simulink model "nonlinearplanner"  (R2021a)
settings: Solver=VariableStepAuto  StartTime=0.0  StopTime=10.0  RelTol=1e-3
values from neighbouring files (symbols this model uses):
  DELAY_LANDING = 4    [variables.m]
  DERIVATIVE_GAIN = 0.002    [variables.m]
  GAIN_LANDING = 0.0022    [variables.m]
  GAIN_TRACK = 0.0038    [variables.m]
  TIME_HOLD = 0.2    [variables.m]
undefined symbols (not defined in the file or in its folder): Ts
libraries: simulink x2
settings Model: Creator=s2130866  LastModifiedBy=s2130866

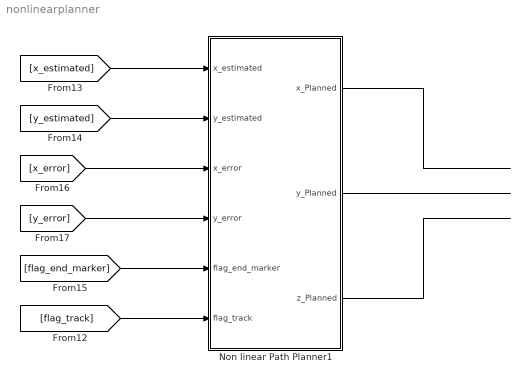
== system nonlinearplanner ==
  Non linear Path Planner1 : Subsystem
  wires:
  Non linear Path Planner1/1(x_Planned) -> ?
  [x_error] -> Non linear Path Planner1/3(x_error)
  Non linear Path Planner1/3(z_Planned) -> ?
  [y_error] -> Non linear Path Planner1/4(y_error)
  [flag_end_marker] -> Non linear Path Planner1/5(flag_end_marker)
  [x_estimated] -> Non linear Path Planner1/1(x_estimated)
  [flag_track] -> Non linear Path Planner1/6(flag_track)
  [y_estimated] -> Non linear Path Planner1/2(y_estimated)
  Non linear Path Planner1/2(y_Planned) -> ?

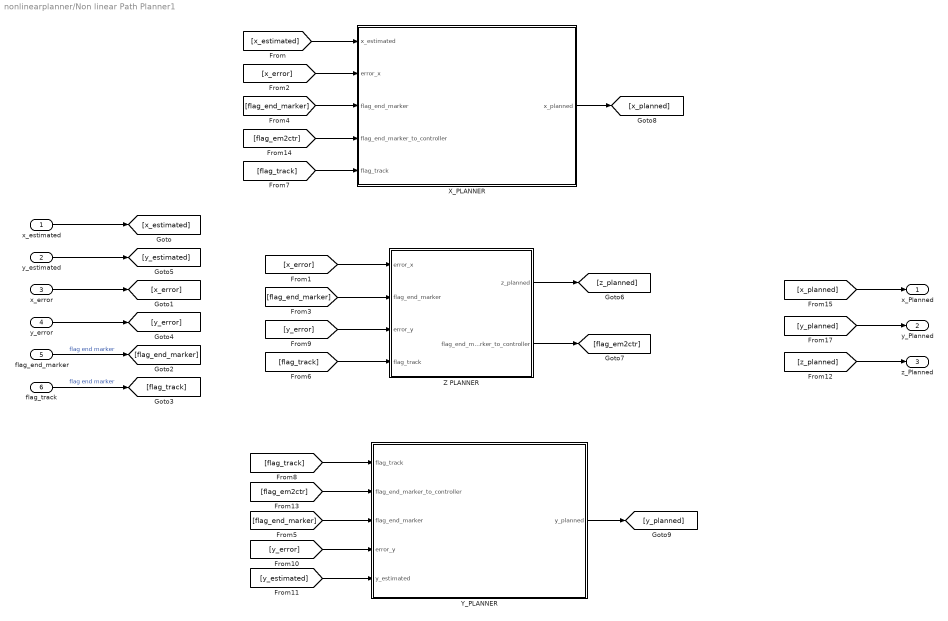
== system nonlinearplanner/Non linear Path Planner1 ==
  x_estimated : Inport
  y_estimated : Inport  Port=2
  x_error : Inport  Port=3
  y_error : Inport  Port=4
  flag_end_marker : Inport  Port=5
  flag_track : Inport  Port=6
  X_PLANNER : Subsystem
  Y_PLANNER : Subsystem
  Z PLANNER : Subsystem
  x_Planned : Outport  VectorParamsAs1DForOutWhenUnconnected=off
  y_Planned : Outport  Port=2  VectorParamsAs1DForOutWhenUnconnected=off
  z_Planned : Outport  Port=3  VectorParamsAs1DForOutWhenUnconnected=off
  wires:
  x_estimated/1 -> [x_estimated]
  [x_estimated] -> X_PLANNER/1(x_estimated)
  x_error/1 -> [x_error]
  [x_error] -> Z PLANNER/1(error_x)
  [x_error] -> X_PLANNER/2(error_x)
  flag_end_marker/1 -> [flag_end_marker]  "flag end marker"
  [flag_end_marker] -> Z PLANNER/2(flag_end_marker)
  [flag_end_marker] -> X_PLANNER/3(flag_end_marker)
  [flag_end_marker] -> Y_PLANNER/3(flag_end_marker)
  flag_track/1 -> [flag_track]  "flag end marker"
  [flag_track] -> Z PLANNER/4(flag_track)
  [flag_track] -> X_PLANNER/5(flag_track)
  [flag_track] -> Y_PLANNER/1(flag_track)
  y_error/1 -> [y_error]
  [y_error] -> Z PLANNER/3(error_y)
  [y_error] -> Y_PLANNER/4(error_y)
  y_estimated/1 -> [y_estimated]
  [y_estimated] -> Y_PLANNER/5(y_estimated)
  [z_planned] -> z_Planned/1
  Z PLANNER/1(z_planned) -> [z_planned]
  Z PLANNER/2(flag_end_marker_to_controller) -> [flag_em2ctr]
  [flag_em2ctr] -> Y_PLANNER/2(flag_end_marker_to_controller)
  [flag_em2ctr] -> X_PLANNER/4(flag_end_marker_to_controller)
  X_PLANNER/1(x_planned) -> [x_planned]
  Y_PLANNER/1(y_planned) -> [y_planned]
  [x_planned] -> x_Planned/1
  [y_planned] -> y_Planned/1

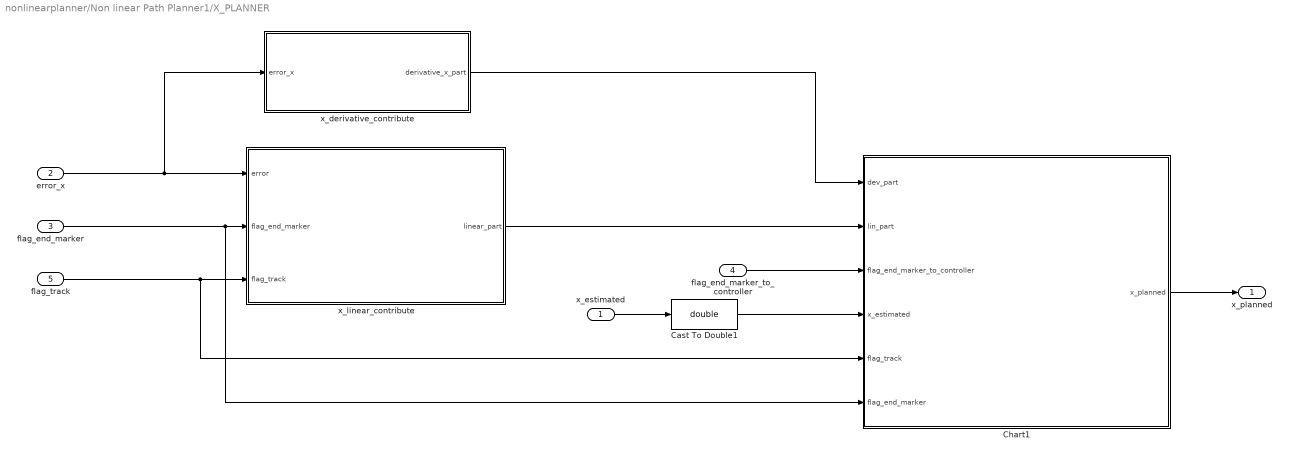
== system nonlinearplanner/Non linear Path Planner1/X_PLANNER ==
  x_estimated : Inport
  error_x : Inport  Port=2
  flag_end_marker : Inport  Port=3
  flag_end_marker_to_controller : Inport  Port=4
  flag_track : Inport  Port=5
  Cast To Double1 : DataTypeConversion  OutDataTypeStr=double
  Chart1 : Stateflow chart  TreatAsAtomicUnit=on
  "x_derivative_contribute " : Subsystem
  x_linear_contribute : Stateflow chart  TreatAsAtomicUnit=on
  x_planned : Outport  VectorParamsAs1DForOutWhenUnconnected=off
  wires:
  "x_derivative_contribute "/1(derivative_x_part) -> Chart1/1(dev_part)
  x_estimated/1 -> Cast To Double1/1
  flag_end_marker_to_controller/1 -> Chart1/3(flag_end_marker_to_controller)
  error_x/1 -> "x_derivative_contribute "/1(error_x), x_linear_contribute/1(error)
  Cast To Double1/1 -> Chart1/4(x_estimated)
  flag_track/1 -> Chart1/5(flag_track), x_linear_contribute/3(flag_track)
  x_linear_contribute/1(linear_part) -> Chart1/2(lin_part)
  flag_end_marker/1 -> Chart1/6(flag_end_marker), x_linear_contribute/2(flag_end_marker)
  Chart1/1(x_planned) -> x_planned/1

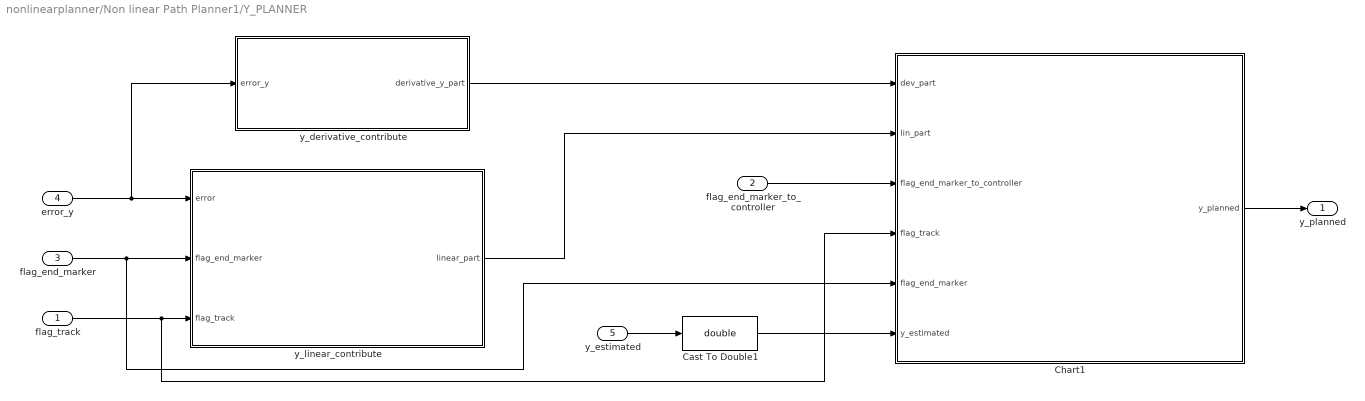
== system nonlinearplanner/Non linear Path Planner1/Y_PLANNER ==
  flag_track : Inport
  flag_end_marker_to_controller : Inport  Port=2
  flag_end_marker : Inport  Port=3
  error_y : Inport  Port=4
  y_estimated : Inport  Port=5
  Cast To Double1 : DataTypeConversion  OutDataTypeStr=double
  Chart1 : Stateflow chart  TreatAsAtomicUnit=on
  "y_derivative_contribute " : Subsystem
  y_linear_contribute : Stateflow chart  TreatAsAtomicUnit=on
  y_planned : Outport  VectorParamsAs1DForOutWhenUnconnected=off
  wires:
  error_y/1 -> y_linear_contribute/1(error), "y_derivative_contribute "/1(error_y)
  "y_derivative_contribute "/1(derivative_y_part) -> Chart1/1(dev_part)
  y_estimated/1 -> Cast To Double1/1
  flag_end_marker/1 -> Chart1/5(flag_end_marker), y_linear_contribute/2(flag_end_marker)
  flag_track/1 -> Chart1/4(flag_track), y_linear_contribute/3(flag_track)
  y_linear_contribute/1(linear_part) -> Chart1/2(lin_part)
  Cast To Double1/1 -> Chart1/6(y_estimated)
  flag_end_marker_to_controller/1 -> Chart1/3(flag_end_marker_to_controller)
  Chart1/1(y_planned) -> y_planned/1

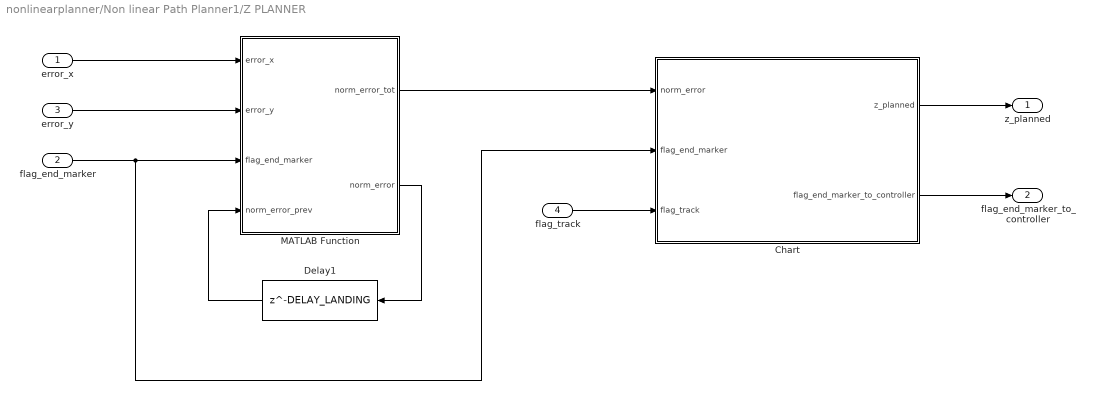
== system nonlinearplanner/Non linear Path Planner1/Z PLANNER ==
  error_x : Inport
  flag_end_marker : Inport  Port=2
  error_y : Inport  Port=3
  flag_track : Inport  Port=4
  Chart : Stateflow chart  TreatAsAtomicUnit=on
  Delay1 : Delay  DelayLength=DELAY_LANDING
  MATLAB Function : MATLAB Function  TreatAsAtomicUnit=on
  z_planned : Outport  VectorParamsAs1DForOutWhenUnconnected=off
  flag_end_marker_to_controller : Outport  Port=2  VectorParamsAs1DForOutWhenUnconnected=off
  wires:
  error_y/1 -> MATLAB Function/2(error_y)
  error_x/1 -> MATLAB Function/1(error_x)
  flag_end_marker/1 -> Chart/2(flag_end_marker), MATLAB Function/3(flag_end_marker)
  MATLAB Function/2(norm_error) -> Delay1/1
  Delay1/1 -> MATLAB Function/4(norm_error_prev)
  MATLAB Function/1(norm_error_tot) -> Chart/1(norm_error)
  Chart/1(z_planned) -> z_planned/1
  flag_track/1 -> Chart/3(flag_track)
  Chart/2(flag_end_marker_to_controller) -> flag_end_marker_to_controller/1

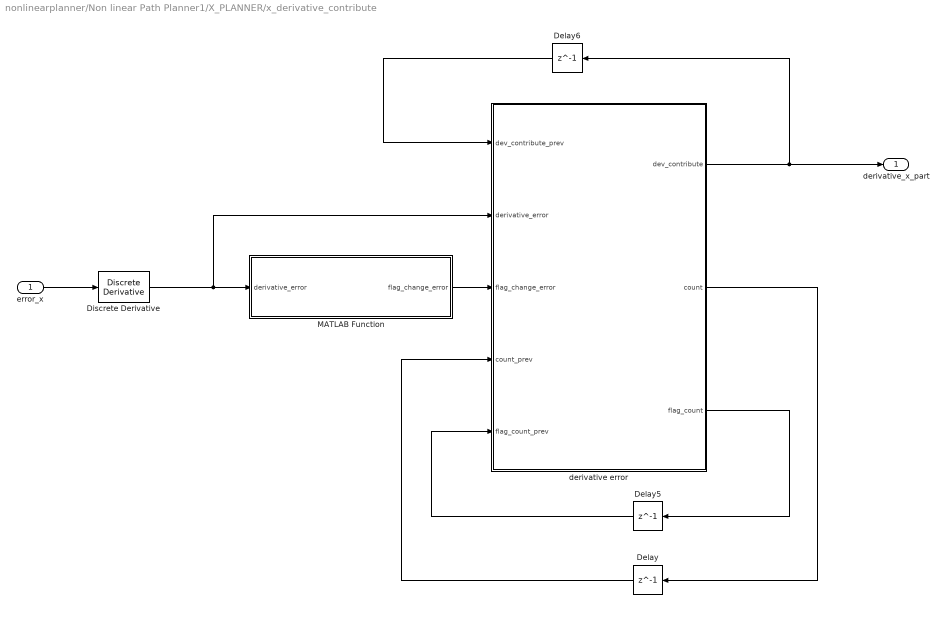
== system nonlinearplanner/Non linear Path Planner1/X_PLANNER/x_derivative_contribute  ==
  error_x : Inport
  Delay : Delay  DelayLength=1  InitialCondition=0
  Delay5 : Delay  DelayLength=1
  Delay6 : Delay  DelayLength=1  InitialCondition=0
  Discrete Derivative : simulink/Discrete/Discrete Derivative  gainval=Ts  ICPrevScaledInput=0.0  OutMin=[]  OutMax=[]  OutDataType=fixdt(1, 16)  OutScaling=2^-10  DoSatur=off
  MATLAB Function : MATLAB Function  TreatAsAtomicUnit=on
  derivative error : MATLAB Function  TreatAsAtomicUnit=on
  derivative_x_part : Outport  VectorParamsAs1DForOutWhenUnconnected=off
  wires:
  error_x/1 -> Discrete Derivative/1
  derivative error/3(flag_count) -> Delay5/1
  derivative error/2(count) -> Delay/1
  Delay/1 -> derivative error/4(count_prev)
  Discrete Derivative/1 -> derivative error/2(derivative_error), MATLAB Function/1(derivative_error)
  Delay5/1 -> derivative error/5(flag_count_prev)
  MATLAB Function/1(flag_change_error) -> derivative error/3(flag_change_error)
  derivative error/1(dev_contribute) -> Delay6/1, derivative_x_part/1
  Delay6/1 -> derivative error/1(dev_contribute_prev)

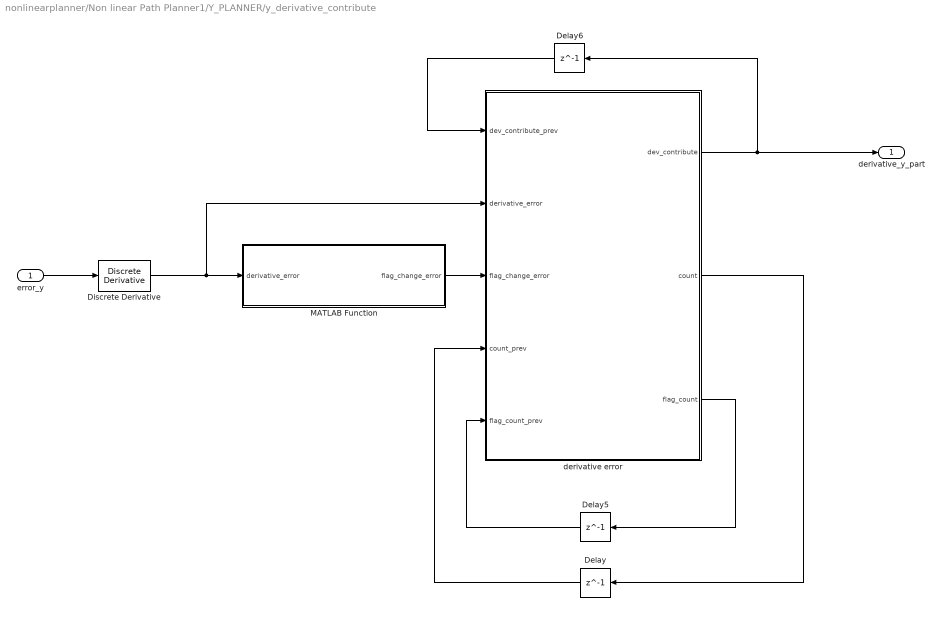
== system nonlinearplanner/Non linear Path Planner1/Y_PLANNER/y_derivative_contribute  ==
  error_y : Inport
  Delay : Delay  DelayLength=1  InitialCondition=0
  Delay5 : Delay  DelayLength=1
  Delay6 : Delay  DelayLength=1  InitialCondition=0
  Discrete Derivative : simulink/Discrete/Discrete Derivative  gainval=Ts  ICPrevScaledInput=0.0  OutMin=[]  OutMax=[]  OutDataType=fixdt(1, 16)  OutScaling=2^-10  DoSatur=off
  MATLAB Function : MATLAB Function  TreatAsAtomicUnit=on
  derivative error : MATLAB Function  TreatAsAtomicUnit=on
  derivative_y_part : Outport  VectorParamsAs1DForOutWhenUnconnected=off
  wires:
  error_y/1 -> Discrete Derivative/1
  derivative error/3(flag_count) -> Delay5/1
  derivative error/2(count) -> Delay/1
  Delay/1 -> derivative error/4(count_prev)
  Discrete Derivative/1 -> derivative error/2(derivative_error), MATLAB Function/1(derivative_error)
  Delay5/1 -> derivative error/5(flag_count_prev)
  MATLAB Function/1(flag_change_error) -> derivative error/3(flag_change_error)
  derivative error/1(dev_contribute) -> Delay6/1, derivative_y_part/1
  Delay6/1 -> derivative error/1(dev_contribute_prev)

== stateflow chart nonlinearplanner/Non linear Path Planner1/Y_PLANNER/Chart1 ==
  state STATE [group]
    - TRACKING: the drone is tracking the lane of the end-marker.
    - LANDING: the drone is landing when the end-marker is dected and the error between the drone CoG and the
    middle point of the end-marker is less than MAX_ERROR_LANDING.
    - TRACK_DETECTED: the Image Processing System detected the lane.
    - END_MARKER_DETECTED: the Image Processing System detected the end-marker.
  state INPUT [group]
    - flag_track: flag raised when the track is detected by Image Processing System.
    - flag_end_marker_to_Controller: flag raised when the drone has to land.
    - lin_part: linear part of the path planner.
    - dev_part: derivative part of the path planner.
    - y_estimated: estimated drone position along the y-axis.
    - flag_end_marker : flag raised when the end-marker is detected by the Image Processing System.
  state OUTPUT [group]
    - y_planned: y coordinate of the goal position.
  state TRACKING
    state TRACK_DETECTED
      during:
      y_planned= y_estimated + lin_part + dev_part;
      y_planned_stored=y_planned;
    state END_MARKER_DETECTED
      during:
      y_planned= y_estimated + lin_part ;
      y_planned_stored=y_planned;
    (default) -> TRACK_DETECTED
    TRACK_DETECTED -> END_MARKER_DETECTED : [flag_end_marker==1 && flag_track==0]
    END_MARKER_DETECTED -> TRACK_DETECTED : [flag_end_marker==0 && flag_track==1]
  state LANDING
    during:
    y_planned=y_planned_stored;
  state IDLE
  (default) -> IDLE
  IDLE -> TRACKING : [flag_track==1 && flag_end_marker==0]
  TRACKING -> LANDING : [flag_end_marker_to_controller==1]
  data: dev_part input double; lin_part input double; flag_end_marker_to_controller input double; flag_track input double; flag_end_marker input double; y_estimated input; y_planned_stored local double; y_planned output double

== matlab function nonlinearplanner/Non linear Path Planner1/Y_PLANNER/y_derivative_contribute /MATLAB Function ==
  data: derivative_error input; flag_change_error output; CHANGE_DERIVATIVE_ERROR_THRESHOLD parameter
function flag_change_error = change_error_checker(derivative_error, ...
    CHANGE_DERIVATIVE_ERROR_THRESHOLD)
% This MATLAB function recognizes if the derivative of the error is greater
% than a threshold value, i.e., the  CHANGE_DERIVATIVE_ERROR_THRESHOLD. 
% 
% Input:
% - derivative_error: derivative of the error. The error is expressed in 
% pixels
%
% Parameter:
% - CHANGE_DERIVATIVE_ERROR_THRESHOLD: threshold value.
%
% Output:
% - flag_change_error: flag raised when the derivative of the error
% changes.

if abs(derivative_error) >= CHANGE_DERIVATIVE_ERROR_THRESHOLD

    flag_change_error = 1;

else

    flag_change_error = 0;

end

== matlab function nonlinearplanner/Non linear Path Planner1/Y_PLANNER/y_derivative_contribute /derivative error ==
  data: dev_contribute_prev input; derivative_error input; flag_change_error input; dev_contribute output; count_prev input; count output; flag_count_prev input; flag_count output; Ts parameter; TIME_HOLD parameter; DERIVATIVE_GAIN parameter
function [dev_contribute, count, flag_count] = derivative_error(dev_contribute_prev, ...
    derivative_error, flag_change_error,count_prev,flag_count_prev, Ts, ...
    TIME_HOLD, DERIVATIVE_GAIN)
% This MATLAB function computes the derivative contribution of the path planner
% for the x coordinate.
%
% Inputs:
% - dev_contribute_prev: previous value derative part of the planner
% - derivative_error: derivative error value.
% - flag_change_error: it is raised when the sign of the error changes
% - count_prev: previous value of the counter. 
%
% Parameters:
% - Ts: sampling Time.
% - TIME_HOLD: time to which the previous value assumed by the derivative
% contribute has to be hold.
% - DERIVATIVE_GAIN: gain used for the derivative contribution.
%
% Output:
% - dev_contribute: derivative contribution of the path planner.
% - count: counter value
% - flag_count: flag raises when the derivate contribute does not more take
% part to the pat planner.

persistent count_to_be_hold

if isempty(count_to_be_hold)
    count_to_be_hold = round(TIME_HOLD/Ts);
end

flag_count = 0;

if flag_change_error && count_prev == 0    
    flag_count=1;   
end
   
if flag_count_prev || flag_count
    
    if count_prev == count_to_be_hold

        count=0;
        flag_count=0;

    else

        count=count_prev+1;
        flag_count=1;
        
    end
    
    dev_contribute=derivative_error*DERIVATIVE_GAIN;
    
    if dev_contribute ==0 && dev_contribute_prev ~=0 
        
        dev_contribute=dev_contribute_prev;
        
    end

else
    
    flag_count = 0;
    count = 0;
    dev_contribute = 0;
    
end

== stateflow chart nonlinearplanner/Non linear Path Planner1/Y_PLANNER/y_linear_contribute ==
  state STATE [group]
    - TRACKING: the drone is tracking the lane or the end-marker.
    - LANDING: the drone lands when the end-marker is detected and the error between the drone CoG and the middle
    of the end-marker is less than MAX_ERROR_LANDING.
    - TRACK_DETECTED: the Image Processing System detected the lane.
    - END_MARKER_DETECTED: the Image Processing System detected the end-marker.
  state INPUT [group]
    - flag_track: flag raised when the lane is detected by Image Processing System.
    - flag_end_marker_to_controller: flag raised when the drone has to land.
    - lin_part: linear part of the path planner.
    - dev_part: derivative part of the path planner.
    - y_estimated: y coordinate of the drone position.
    - flag_end_marker: flag raised when the end-marker is detected by Image Processing System.
  state PARAMETERS [group]
    - GAIN_TRACK: gain used by the drone reference generator to follow the lane.
    - GAIN_LANDING: gain used by the drone reference generator to land over the end-marker.
  state OUTPUT [group]
    - y_planned: y coordinate of the goal position.
  state END_MARKER_DETECTED
    during:
    linear_part = error * GAIN_LANDING;
  state IDLE
  state TRACK_DETECTED
    during:
    linear_part = error * GAIN_TRACK;
  TRACK_DETECTED -> END_MARKER_DETECTED : [flag_end_marker==1 && flag_track==0]
  IDLE -> TRACK_DETECTED : [flag_end_marker==0 && flag_track==1]
  (default) -> IDLE
  data: error input double; GAIN_TRACK parameter double; GAIN_LANDING parameter double; flag_end_marker input double; flag_track input double; linear_part output double

== stateflow chart nonlinearplanner/Non linear Path Planner1/Z PLANNER/Chart ==
  state STATE [group]
    - TRACKING: The drone is tracking the lane or the end-marker when they are detected.
    - LANDING: The drone is landing when the land-marker is detected and the error between the drone CoG and
    the central point of the end-marker is less than MAX_ERROR_LANDING.
  state INPUT [group]
    - flag_track: flag raised when the lane is detected by the Image Processing System.
    - flag_end_marker: flag raised when the end-marker is detected by the Image Processing System.
    - norm error: error between the drone CoG and the central point of the end-marker.
  state OUTPUT [group]
    - z_planned: drone altitude sent to the drone controller.
    - flag_end_marker_to_controller: flag raise when the drone has to land.
  state TRACKING
    entry:
    z_planned =  -1.1 ;
    flag_end_marker_to_controller=0;
  state LANDING
    entry:
    z_planned =  0 ;
    flag_end_marker_to_controller=1;
  state IDLE
    entry:
    z_planned =  -1.1 ;
    flag_end_marker_to_controller=0;
  (default) -> IDLE
  IDLE -> TRACKING : [flag_track==1]
  TRACKING -> LANDING : [flag_end_marker==1 && norm_error <= MAX_ERROR_LANDING]
  data: norm_error input double; z_planned output double; MAX_ERROR_LANDING parameter double; flag_end_marker input; flag_track input; flag_end_marker_to_controller output double

== matlab function nonlinearplanner/Non linear Path Planner1/Z PLANNER/MATLAB Function ==
  data: norm_error_tot output; error_x input; norm_error output; error_y input; flag_end_marker input; norm_error_prev input
function [norm_error_tot, norm_error] = error_function(error_x, error_y, ...
flag_end_marker, norm_error_prev)
% This MATLAB function computes the norm of the error between the drone CoG
% drone and the middle of point of the end-marker. The norm error is
% computed only if the end-marker is detected.
%
%
%Inputs:
% - error_x: error along the x-axis between the drone CoG and the central 
% point of the end-marker.
% - error_y: error along the y-axis between the drone CoG and the central 
% point of the end-marker.
% - flag_end_marker: the flag indicates when the end-marker is detected.
% - norm_error_prev: previous value of the norm of the error.                                                                                                                                              
%  
%
%Outputs:
% - norm_error_tot: norm of the error between the drone CoG and the central 
% point of the end-marker. It consideres the previous value assumed by the
% norm of the error. The values is condisder at the time k = time_step +
% DELAY_LANDING \cdot sampling time. 
% - norm_error: actual value assumed by the norm of error. The error is 
% computed by the drone CoG and the middle point of the end-marker.

if flag_end_marker
    
    norm_error = sqrt((error_x)^2 + (error_y)^2);
    norm_error_tot = norm_error + norm_error_prev  ;
    
else 
    %100 is a constant value greater than MAX_ERROR_LANDING
    norm_error_tot = 100;
    norm_error = 100;
end

== stateflow chart nonlinearplanner/Non linear Path Planner1/X_PLANNER/Chart1 ==
  state STATE [group]
    - TRACKING: The drone is tracking the lane or the end-marker.
    - LANDING: The drone is landing if the end-marker is detected and the error between the drone CoG and the middle
    point of the end-marker is less than MAX_ERROR_LANDING.
    - TRACK_DETECTED: The Image Processing System detected the lane.
    - END_MARKER_DETECTED: The Image Processing System detected the end-marker.
  state INPUT [group]
    - flag_track: flag raised when the track is detected by the Image Processing System.
    - flag_end_marker_to_controller: flag raised when the drone has to land.
    - lin_part: linear part of the path planner.
    - dev_part: derivative part of the path planner.
    - x_estimated: postion x estimated from the sensors.
    - flag_end_marker: flag raised when the land-marker is detected by the Image Processing System.
  state OUTPUT [group]
    - x_planned: x coordinate of the goal position.
  state TRACKING
    state TRACK_DETECTED
      during:
      x_planned = x_estimated + lin_part + dev_part;
      x_planned_stored = x_planned;
    state END_MARKER_DETECTED
      during:
      x_planned = x_estimated + lin_part ;
      x_planned_stored = x_planned;
    (default) -> TRACK_DETECTED
    TRACK_DETECTED -> END_MARKER_DETECTED : [flag_end_marker==1 && flag_track==0]
    END_MARKER_DETECTED -> TRACK_DETECTED : [flag_end_marker==0 && flag_track==1]
  state LANDING
    during:
    x_planned=x_planned_stored;
  state IDLE
  (default) -> IDLE
  IDLE -> TRACKING : [flag_track==1 && flag_end_marker==0]
  TRACKING -> LANDING : [flag_end_marker_to_controller==1]
  data: dev_part input double; lin_part input double; x_planned output double; flag_end_marker_to_controller input double; x_estimated input double; flag_track input double; x_planned_stored local double; flag_end_marker input double

== matlab function nonlinearplanner/Non linear Path Planner1/X_PLANNER/x_derivative_contribute /MATLAB Function ==
  data: derivative_error input; flag_change_error output; CHANGE_DERIVATIVE_ERROR_THRESHOLD parameter
function flag_change_error = change_error_checker(derivative_error, ...
    CHANGE_DERIVATIVE_ERROR_THRESHOLD)
% This MATLAB function recognizes if the derivative of the error is greater
% than a threshold value, i.e., the  CHANGE_DERIVATIVE_ERROR_THRESHOLD. 
% 
% Input:
% - derivative_error: derivative of the error. The error is expressed in 
% pixels
%
% Parameter:
% - CHANGE_DERIVATIVE_ERROR_THRESHOLD: threshold value.
%
% Output:
% - flag_change_error: flag raised when the derivative of the error
% changes.

if abs(derivative_error) >= CHANGE_DERIVATIVE_ERROR_THRESHOLD

    flag_change_error = 1;

else

    flag_change_error = 0;

end

== matlab function nonlinearplanner/Non linear Path Planner1/X_PLANNER/x_derivative_contribute /derivative error ==
  data: dev_contribute_prev input; derivative_error input; flag_change_error input; dev_contribute output; count_prev input; count output; flag_count_prev input; flag_count output; Ts parameter; TIME_HOLD parameter; DERIVATIVE_GAIN parameter
function [dev_contribute, count, flag_count] = derivative_error(dev_contribute_prev, ...
    derivative_error, flag_change_error,count_prev,flag_count_prev, Ts, ...
    TIME_HOLD, DERIVATIVE_GAIN)
% This MATLAB function computes the derivative contribution of the path planner
% for the x coordinate.
%
% Inputs:
% - dev_contribute_prev: previous value derative part of the planner
% - derivative_error: derivative error value.
% - flag_change_error: it is raised when the sign of the error changes
% - count_prev: previous value of the counter. 
%
% Parameters:
% - Ts: sampling Time.
% - TIME_HOLD: time to which the previous value assumed by the derivative
% contribute has to be hold.
% - DERIVATIVE_GAIN: gain used for the derivative contribution.
%
% Output:
% - dev_contribute: derivative contribution of the path planner.
% - count: counter value
% - flag_count: flag raises when the derivate contribute does not more take
% part to the pat planner.

persistent count_to_be_hold

if isempty(count_to_be_hold)
    count_to_be_hold = round(TIME_HOLD/Ts);
end

flag_count = 0;

if flag_change_error && count_prev == 0    
    flag_count=1;   
end
   
if flag_count_prev || flag_count
    
    if count_prev == count_to_be_hold

        count=0;
        flag_count=0;

    else

        count=count_prev+1;
        flag_count=1;
        
    end
    
    dev_contribute=derivative_error*DERIVATIVE_GAIN;
    
    if dev_contribute ==0 && dev_contribute_prev ~=0 
        
        dev_contribute=dev_contribute_prev;
        
    end

else
    
    flag_count = 0;
    count = 0;
    dev_contribute = 0;
    
end

== stateflow chart nonlinearplanner/Non linear Path Planner1/X_PLANNER/x_linear_contribute ==
  state STATE [group]
    - TRACK_DETECTED: The Image Processing System detected the lane.
    - END_MARKER_DETECTED: The Image Processing System detected the end-marker.
  state INPUT [group]
    - Flag_track: flag raised when the lane is detected by the Image Processing System.
    - Flag_end_marker : flag raised when the end-marker is detected by the Image Processing System.
  state PARAMETERS [group]
    - GAIN_TRACK: gain used from the drone reference generator when it follows the lane.
    - GAIN_LANDING: gain used from the drone reference generator for landing on the end-marker.
  state OUTPUT [group]
    - linear_part : linear contribute.
  state END_MARKER_DETECTED
    during:
    linear_part = error * GAIN_LANDING;
  state IDLE
  state TRACK_DETECTED
    during:
    linear_part = error * GAIN_TRACK;
  TRACK_DETECTED -> END_MARKER_DETECTED : [flag_end_marker==1 && flag_track==0]
  IDLE -> TRACK_DETECTED : [flag_end_marker==0 && flag_track==1]
  (default) -> IDLE
  data: error input double; GAIN_TRACK parameter double; GAIN_LANDING parameter double; flag_end_marker input double; flag_track input double; linear_part output double
